simulink model "pid_based_model_2"  (R2021a)
settings: Solver=VariableStepAuto  StartTime=0.0  StopTime=300  RelTol=1e-3
libraries: pid_lib x1
settings Model: Creator=uddin  LastModifiedBy=uddin

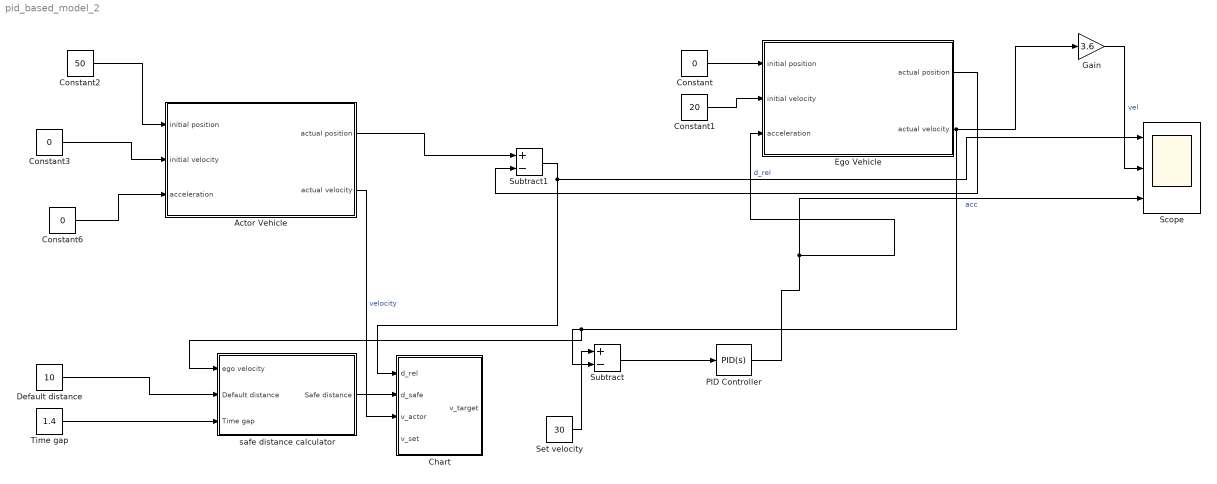
== system pid_based_model_2 ==
  Actor Vehicle : Subsystem
  Chart : Stateflow chart  TreatAsAtomicUnit=on
  Constant : Constant  Value=0  SampleTime=-1
  Constant1 : Constant  Value=20  SampleTime=-1
  Constant2 : Constant  Value=50  SampleTime=-1
  Constant3 : Constant  Value=0  SampleTime=-1
  Constant6 : Constant  Value=0  SampleTime=-1
  Default distance : Constant  Value=10  SampleTime=.1
  Ego Vehicle : Subsystem
  Gain : Gain  Gain=3.6
  PID Controller : pid_lib/PID Controller  Controller=PID  Form=Parallel  TimeDomain=Continuous-time  UseExternalTs=off  SampleTime=-1  IntegratorMethod=Forward Euler  FilterMethod=Forward Euler  ControllerParametersSource=internal  P=30.0672634232495  I=7.64046491440372  D=17.8175411585063  UseFilter=on  N=4070.78873884721  TunerSelectOption=Transfer Function Based (PID Tuner App)  InitialConditionSource=internal  InitialConditionForIntegrator=0  InitialConditionForFilter=0  DifferentiatorICPrevScaledInput=0  ExternalReset=none  TrackingMode=off  Kt=1  LimitOutput=on  SatLimitsSource=internal  UpperSaturationLimit=inf  LowerSaturationLimit=-inf  LinearizeAsGain=on  AntiWindupMode=none  Kb=1  POutMin=[]  POutMax=[]  IOutMin=[]  IOutMax=[]  DOutMin=[]  DOutMax=[]  NOutMin=[]  NOutMax=[]  SumOutMin=[]  SumOutMax=[]  SaturationOutMin=[]  SaturationOutMax=[]  PParamMin=[]  PParamMax=[]  IParamMin=[]  IParamMax=[]  DParamMin=[]  DParamMax=[]  NParamMin=[]  NParamMax=[]  KbParamMin=[]  KbParamMax=[]  KtParamMin=[]  KtParamMax=[]  KbOutMin=[]  KbOutMax=[]  KtOutMin=[]  KtOutMax=[]  IntegratorOutMin=[]  IntegratorOutMax=[]  FilterOutMin=[]  FilterOutMax=[]  SumI1OutMin=[]  SumI1OutMax=[]  SumI2OutMin=[]  SumI2OutMax=[]  SumI3OutMin=[]  SumI3OutMax=[]  SumI4OutMin=[]  SumI4OutMax=[]  SumDOutMin=[]  SumDOutMax=[]  DifferentiatorOutMin=[]  DifferentiatorOutMax=[]  FilterDiffOutCoefMin=[]  FilterDiffOutCoefMax=[]  ReciprocalOutMin=[]  ReciprocalOutMax=[]  SumDenOutMin=[]  SumDenOutMax=[]  SumNumOutMin=[]  SumNumOutMax=[]  DivideOutMin=[]  DivideOutMax=[]  UdiffTsProdOutMin=[]  UdiffTsProdOutMax=[]  NTsProdOutMin=[]  NTsProdOutMax=[]  UintegralTsProdOutMin=[]  UintegralTsProdOutMax=[]  UngainTsProdOutMin=[]  UngainTsProdOutMax=[]  IntegratorContinuousStateAttributes=''  IntegratorStateMustResolveToSignalObject=off  IntegratorRTWStateStorageClass=Auto  FilterContinuousStateAttributes=''  FilterStateMustResolveToSignalObject=off  FilterRTWStateStorageClass=Auto  ParallelPVariant=InternalParameters  IdealPVariant=Disabled  IVariant=InternalParameters  DVariant=InternalParameters  IntegratorVariant=Continuous  SatVariant=Enabled  AWVariant=Passthrough  PCopyVariant=Disabled  TRVariant=Disabled  FdbkBlocksVariant=Forward  IdealPFdbkVariant=Disabled  SatFdbkVariant=Disabled  DerivativeFilterVariant=ContFilter  NVariant=InternalParameters  NCopyVariant=Disabled  FilterICVariant=InternalICsFilter  IntegratorICVariant=InternalICs  ExternalResetVariant=Disabled  TRSumVariant=Passthrough  SumFdbkVariant=Disabled  SumVariant=Sum_PID  TsampFilterVariant=InternalTs  TsampNgainVariant=Passthrough  TsampIntegralVariant=Passthrough  ExternalSaturationOutDataTypeStr=Inherit: Same as second input
  Scope : Scope  NumInputPorts=3
  Set velocity : Constant  Value=30  SampleTime=.1
  Subtract : Sum  Inputs=+-
  Subtract1 : Sum  Inputs=+-
  Time gap : Constant  Value=1.4  SampleTime=.1
  safe distance calculator : Subsystem
  wires:
  Constant2/1 -> Actor Vehicle/1(initial position)
  Constant6/1 -> Actor Vehicle/3(acceleration)
  Constant3/1 -> Actor Vehicle/2(initial velocity)
  Constant/1 -> Ego Vehicle/1(initial position)
  Constant1/1 -> Ego Vehicle/2(initial velocity)
  Ego Vehicle/2(actual velocity) -> safe distance calculator/1(ego velocity), Subtract/2, Gain/1
  Gain/1 -> Scope/2  "vel"
  Default distance/1 -> safe distance calculator/2(Default distance)
  Time gap/1 -> safe distance calculator/3(Time gap)
  Ego Vehicle/1(actual position) -> Subtract1/2
  Subtract1/1 -> Scope/1, Chart/1(d_rel)  "d_rel"
  safe distance calculator/1(Safe distance) -> Chart/2(d_safe)
  Actor Vehicle/1(actual position) -> Subtract1/1
  Actor Vehicle/2(actual velocity) -> Chart/3(v_actor)  "velocity"
  PID Controller/1 -> Ego Vehicle/3(acceleration), Scope/3  "acc"
  Subtract/1 -> PID Controller/1
  Set velocity/1 -> Subtract/1

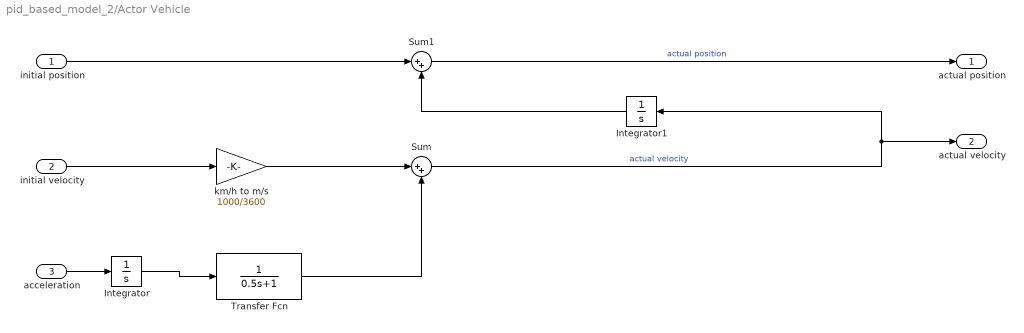
== system pid_based_model_2/Actor Vehicle ==
  initial position : Inport
  initial velocity : Inport  Port=2
  acceleration : Inport  Port=3
  Integrator : Integrator
  Integrator1 : Integrator
  Sum : Sum  Inputs=|++
  Sum1 : Sum  Inputs=|++
  Transfer Fcn : TransferFcn  Denominator=[0.5 1]
  km/h to m/s : Gain  Gain=1000/3600
  actual position : Outport
  actual velocity : Outport  Port=2
  wires:
  km/h to m/s/1 -> Sum/1
  initial velocity/1 -> km/h to m/s/1
  Transfer Fcn/1 -> Sum/2
  Integrator/1 -> Transfer Fcn/1
  Integrator1/1 -> Sum1/2
  initial position/1 -> Sum1/1
  acceleration/1 -> Integrator/1
  Sum/1 -> Integrator1/1, actual velocity/1  "actual velocity"
  Sum1/1 -> actual position/1  "actual position"

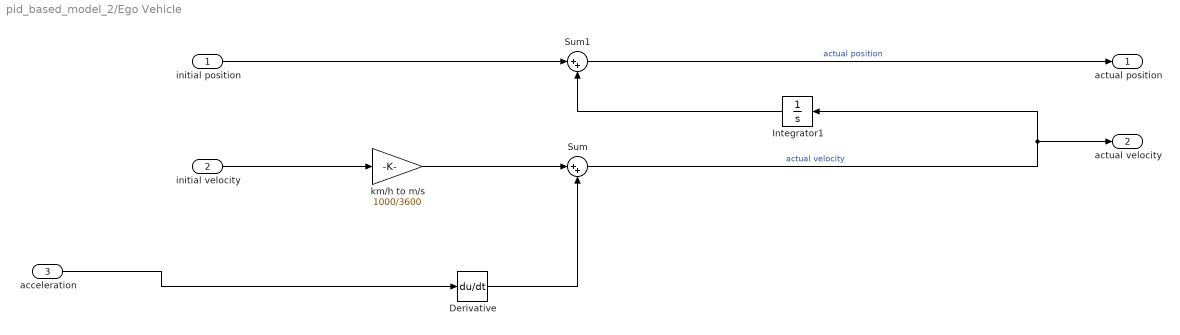
== system pid_based_model_2/Ego Vehicle ==
  initial position : Inport
  initial velocity : Inport  Port=2
  acceleration : Inport  Port=3
  Derivative : Derivative
  Integrator1 : Integrator
  Sum : Sum  Inputs=|++
  Sum1 : Sum  Inputs=|++
  km/h to m/s : Gain  Gain=1000/3600
  actual position : Outport
  actual velocity : Outport  Port=2
  wires:
  Sum1/1 -> actual position/1  "actual position"
  Sum/1 -> actual velocity/1, Integrator1/1  "actual velocity"
  initial position/1 -> Sum1/1
  Integrator1/1 -> Sum1/2
  initial velocity/1 -> km/h to m/s/1
  km/h to m/s/1 -> Sum/1
  Derivative/1 -> Sum/2
  acceleration/1 -> Derivative/1

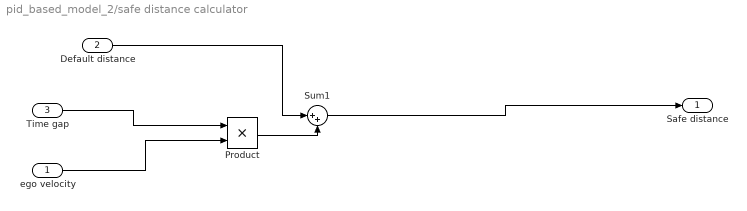
== system pid_based_model_2/safe distance calculator ==
  ego velocity : Inport
  Default distance : Inport  Port=2
  Time gap : Inport  Port=3
  Product : Product
  Sum1 : Sum  Inputs=|++
  Safe distance : Outport
  wires:
  Product/1 -> Sum1/2
  Sum1/1 -> Safe distance/1
  Time gap/1 -> Product/1
  ego velocity/1 -> Product/2
  Default distance/1 -> Sum1/1

== stateflow chart pid_based_model_2/Chart ==
  (default) -> (junction 7)
  (junction 7) -> (junction 8) [order 1] : [d_rel>=d_safe]
  (junction 7) -> (junction 9) [order 2] : {v_target=v_actor;}
  (junction 8) -> (junction 10) : {v_target=v_set;}
  (junction 10) -> (junction 9)
  (junction 9) -> (junction 11)
  data: d_rel input; d_safe input; v_actor input; v_set input; v_target output
